simulink model "voiceActivityDet_ver"  (R2019a)
settings: Solver=VariableStepAuto  StartTime=0.0  StopTime=(nSamp-1)*Ts  RelTol=1e-3
InitFcn:
  | block_verScript;
values from neighbouring files (symbols this model uses):
  FFT_size = 64    [FIR_filterTestm.m]    (also in JMAP_INIT.m; blockVerification.m; block_verScript.m; ksi_verScript.m)
  Ts = 1/Fs    (= 2.08333333333e-05)    [FIR_filterTestm.m]    (also in JMAP_INIT.m; blockVerification.m; block_verScript.m; ksi_verScript.m)
libraries: simulink x2
settings Model: Creator=Showi  LastModifiedBy=Showi

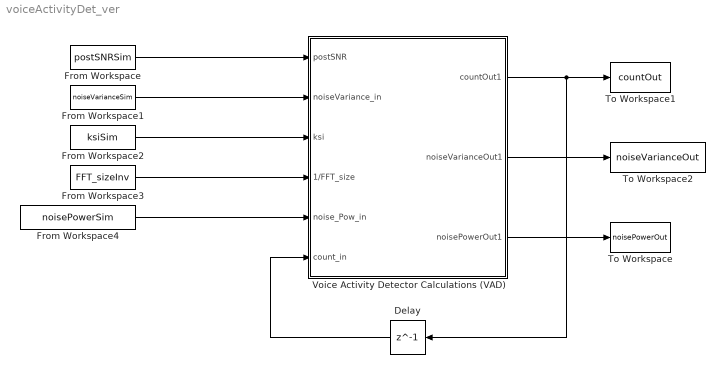
== system voiceActivityDet_ver ==
  Delay : Delay  DelayLength=1  InitialCondition=0  SampleTime=Ts
  From Workspace : FromWorkspace  VariableName=postSNRSim  SampleTime=Ts
  From Workspace1 : FromWorkspace  VariableName=noiseVarianceSim  SampleTime=Ts
  From Workspace2 : FromWorkspace  VariableName=ksiSim  SampleTime=Ts
  From Workspace3 : FromWorkspace  VariableName=FFT_sizeInv  SampleTime=Ts
  From Workspace4 : FromWorkspace  VariableName=noisePowerSim  SampleTime=Ts
  To Workspace : ToWorkspace  VariableName=noisePowerOut  SaveFormat=Structure With Time  SampleTime=Ts
  To Workspace1 : ToWorkspace  VariableName=countOut  SaveFormat=Timeseries  SampleTime=Ts
  To Workspace2 : ToWorkspace  VariableName=noiseVarianceOut  SaveFormat=Structure With Time  SampleTime=Ts
  Voice Activity Detector Calculations (VAD) : Subsystem
  wires:
  From Workspace4/1 -> Voice Activity Detector Calculations (VAD)/5("noise_Pow_in ")
  From Workspace3/1 -> Voice Activity Detector Calculations (VAD)/4(1/FFT_size)
  From Workspace1/1 -> Voice Activity Detector Calculations (VAD)/2(noiseVariance_in)
  From Workspace/1 -> Voice Activity Detector Calculations (VAD)/1(postSNR)
  From Workspace2/1 -> Voice Activity Detector Calculations (VAD)/3(ksi)
  Voice Activity Detector Calculations (VAD)/1(countOut1) -> Delay/1, To Workspace1/1
  Voice Activity Detector Calculations (VAD)/2(noiseVarianceOut1) -> To Workspace2/1
  Voice Activity Detector Calculations (VAD)/3(noisePowerOut1) -> To Workspace/1
  Delay/1 -> Voice Activity Detector Calculations (VAD)/6(count_in)

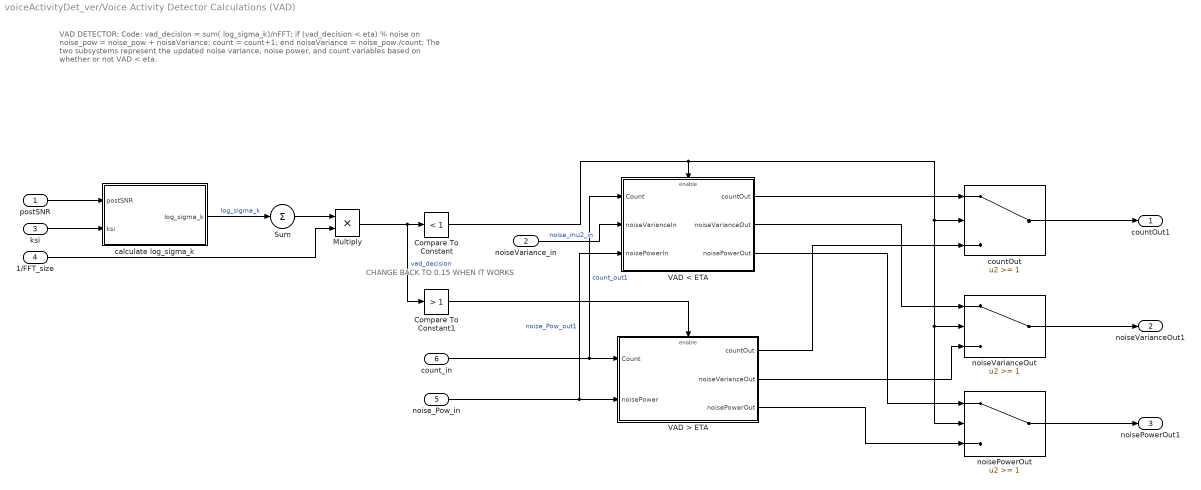
== system voiceActivityDet_ver/Voice Activity Detector Calculations (VAD) ==
  note: VAD DETECTOR:
      |
      | Code:
      |     vad_decision = sum( log_sigma_k)/nFFT;
      |     if (vad_decision < eta) % noise on
      |         noise_pow = noise_pow + noiseVariance;
      |         count = count+1;
      |     end
      |     noiseVariance = noise_pow./count;
      |
      | The two subsystems represent the updated noise variance, noise power, and count variables based
      | on whether or not VAD < eta.
  note: CHANGE BACK TO 0.15 WHEN IT WORKS
  postSNR : Inport
  noiseVariance_in : Inport  Port=2
  ksi : Inport  Port=3
  1/FFT_size : Inport  Port=4
  "noise_Pow_in " : Inport  Port=5
  count_in : Inport  Port=6
  Compare To Constant : simulink/Logic and Bit Operations/Compare To Constant  relop=<  const=1  OutDataTypeStr=boolean
  Compare To Constant1 : simulink/Logic and Bit Operations/Compare To Constant  relop=>  const=1  OutDataTypeStr=boolean
  Multiply : Product  Inputs=**  SaturateOnIntegerOverflow=on  RndMeth=Zero
  Sum : Sum  Inputs=+
  VAD < ETA : Subsystem  TreatAsAtomicUnit=on
  VAD > ETA : Subsystem
  calculate log_sigma_k : Subsystem
  countOut : Switch  Threshold=1
  noisePowerOut : Switch  Threshold=1
  noiseVarianceOut : Switch  Threshold=1
  countOut1 : Outport  InitialOutput=0
  noiseVarianceOut1 : Outport  Port=2  InitialOutput=0
  noisePowerOut1 : Outport  Port=3  InitialOutput=0
  wires:
  postSNR/1 -> calculate log_sigma_k/1(postSNR)
  ksi/1 -> calculate log_sigma_k/2(ksi)
  calculate log_sigma_k/1(log_sigma_k) -> Sum/1  "log_sigma_k"
  Sum/1 -> Multiply/1
  1/FFT_size/1 -> Multiply/2
  Multiply/1 -> Compare To Constant1/1, Compare To Constant/1  "vad_decision"
  "noise_Pow_in "/1 -> VAD < ETA/3(noisePowerIn), VAD > ETA/2(noisePower)  "noise_Pow_out1"
  count_in/1 -> VAD > ETA/1(Count), VAD < ETA/1(Count)  "count_out1"
  Compare To Constant1/1 -> VAD > ETA/Enable
  Compare To Constant/1 -> noisePowerOut/2, noiseVarianceOut/2, countOut/2, VAD < ETA/Enable
  VAD > ETA/1(countOut) -> countOut/3
  VAD > ETA/2(noiseVarianceOut) -> noiseVarianceOut/3
  VAD > ETA/3(noisePowerOut) -> noisePowerOut/3
  VAD < ETA/1(countOut) -> countOut/1
  VAD < ETA/2(noiseVarianceOut) -> noiseVarianceOut/1
  VAD < ETA/3(noisePowerOut) -> noisePowerOut/1
  noiseVariance_in/1 -> VAD < ETA/2(noiseVarianceIn)  "noise_mu2_in"
  noisePowerOut/1 -> noisePowerOut1/1
  noiseVarianceOut/1 -> noiseVarianceOut1/1
  countOut/1 -> countOut1/1

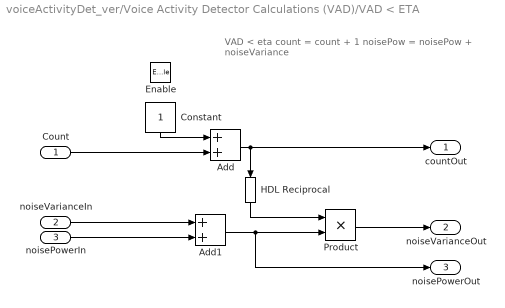
== system voiceActivityDet_ver/Voice Activity Detector Calculations (VAD)/VAD < ETA ==
  note: VAD < eta
      |
      | count = count + 1
      | noisePow = noisePow + noiseVariance
  Count : Inport
  noiseVarianceIn : Inport  Port=2
  noisePowerIn : Inport  Port=3
  Enable : EnablePort
  Add : Sum
  Add1 : Sum
  Constant : Constant  SampleTime=-1
  HDL Reciprocal : Reciprocal
  Product : Product
  countOut : Outport  InitialOutput=0
  noiseVarianceOut : Outport  Port=2  InitialOutput=0
  noisePowerOut : Outport  Port=3  InitialOutput=0
  wires:
  Constant/1 -> Add/1
  Count/1 -> Add/2
  Add/1 -> countOut/1, HDL Reciprocal/1
  noisePowerIn/1 -> Add1/2
  noiseVarianceIn/1 -> Add1/1
  Add1/1 -> noisePowerOut/1, Product/2
  Product/1 -> noiseVarianceOut/1
  HDL Reciprocal/1 -> Product/1

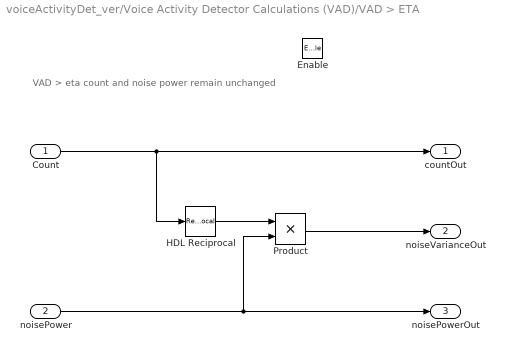
== system voiceActivityDet_ver/Voice Activity Detector Calculations (VAD)/VAD > ETA ==
  note: VAD > eta
      |
      | count and noise power remain unchanged
  Count : Inport
  noisePower : Inport  Port=2
  Enable : EnablePort
  HDL Reciprocal : Reciprocal
  Product : Product
  countOut : Outport
  noiseVarianceOut : Outport  Port=2
  noisePowerOut : Outport  Port=3
  wires:
  Count/1 -> countOut/1, HDL Reciprocal/1
  noisePower/1 -> Product/2, noisePowerOut/1
  Product/1 -> noiseVarianceOut/1
  HDL Reciprocal/1 -> Product/1

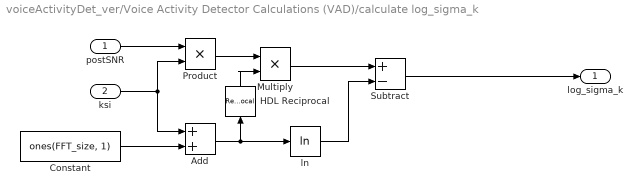
== system voiceActivityDet_ver/Voice Activity Detector Calculations (VAD)/calculate log_sigma_k ==
  postSNR : Inport
  ksi : Inport  Port=2
  Add : Sum
  Constant : Constant  Value=ones(FFT_size, 1)  SampleTime=-1
  HDL Reciprocal : Reciprocal
  Multiply : Product  Inputs=**  SaturateOnIntegerOverflow=on  RndMeth=Zero
  Product : Product
  Subtract : Sum  Inputs=+-
  ln : Math  Operator=log  SaturateOnIntegerOverflow=on
  log_sigma_k : Outport
  wires:
  ksi/1 -> Add/1, Product/2
  Constant/1 -> Add/2
  postSNR/1 -> Product/1
  Product/1 -> Multiply/1
  Add/1 -> HDL Reciprocal/1, ln/1
  Multiply/1 -> Subtract/1
  Subtract/1 -> log_sigma_k/1
  ln/1 -> Subtract/2
  HDL Reciprocal/1 -> Multiply/2
